simulink model "SSV_1"  (R2024a)
settings: Solver=VariableStepAuto  StartTime=0.0  StopTime=10.0  RelTol=1e-6
settings Model: Creator=lenovo  LastModifiedBy=lenovo

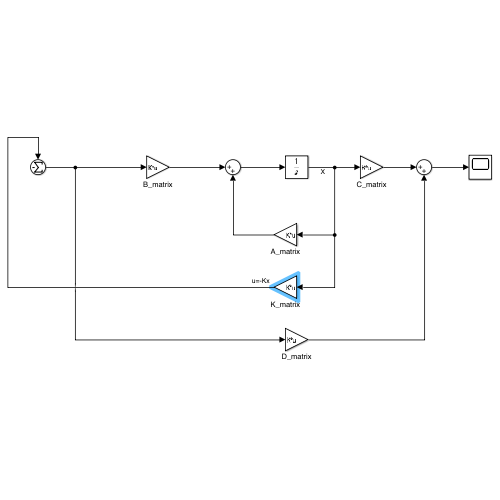
[thumbnail: Simulink's stored preview of the top-level diagram]
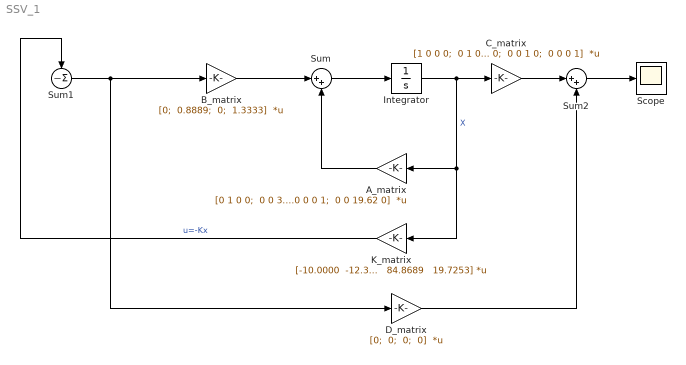
== system SSV_1 ==
  A_matrix : Gain  Gain=|  Multiplication=Matrix(K*u)
      | [0 1 0 0;
      |  0 0 3.27 0;
      |  0 0 0 1;
      |  0 0 19.62 0]
  B_matrix : Gain  Gain=|  Multiplication=Matrix(K*u)
      | [0;
      |  0.8889;
      |  0;
      |  1.3333]
  C_matrix : Gain  Gain=|  Multiplication=Matrix(K*u)
      | [1 0 0 0;
      |  0 1 0 0;
      |  0 0 1 0;
      |  0 0 0 1]
  D_matrix : Gain  Gain=|  Multiplication=Matrix(K*u)
      | [0;
      |  0;
      |  0;
      |  0]
  Integrator : Integrator  InitialCondition=[0.2;0;0.2;0]
  K_matrix : Gain  Gain="[-10.0000  -12.3700   84.8689   19.7253]"  Multiplication=Matrix(K*u)
  Scope : Scope
  Sum : Sum  Inputs=|++
  Sum1 : Sum  Inputs=-|
  Sum2 : Sum  Inputs=|++
  wires:
  Sum/1 -> Integrator/1
  Integrator/1 -> A_matrix/1, K_matrix/1, C_matrix/1  "X"
  A_matrix/1 -> Sum/2
  B_matrix/1 -> Sum/1
  Sum1/1 -> D_matrix/1, B_matrix/1
  C_matrix/1 -> Sum2/1
  D_matrix/1 -> Sum2/2
  Sum2/1 -> Scope/1
  K_matrix/1 -> Sum1/1  "u=-Kx"
